simulink model "13_Solor_Charging_2W"  (R2024a)
settings: Solver=ode23t  StartTime=0.0  StopTime=3600  RelTol=1e-3
undefined symbols (not defined in the file): Ion, Lithium
libraries: spsDiodeLib x2, spsBatteryLib x1, spsSeriesRLCBranchLib x1, spsBoostConverterLib x1, spsParallelRLCBranchLib x1, spsPVArrayLib x1, spspowerguiLib x1
(part 2 of 2)

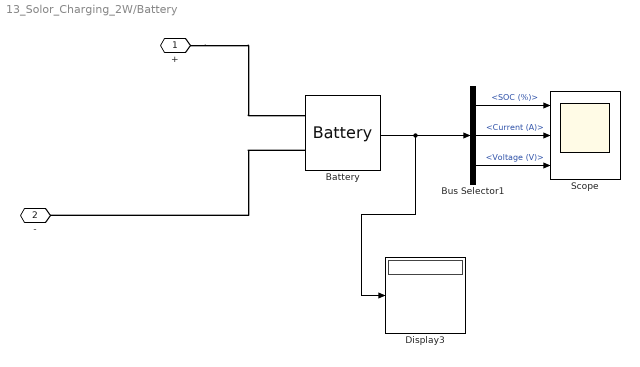
== system 13_Solor_Charging_2W/Battery ==
  Battery : spsBatteryLib/Battery  BatType=Lithium-Ion  ShowTempParam=off  ThermalPreset=no  ShowAgeParam=off  NomV=48  NomQ=65  SOC=25  Batt_Tr=30  PresetModel=on  MaxQ=65  MinV=36  FullV=55.8714  Dis_rate=28.2609  R=0.0073846  Normal_OP=58.7826  expZone="[51.8585      3.19348]"  current=[6.5 13 32.5]  Units=Time  Tci=20  NomT=20  T2=-30  MaxQ2=4.8  FullV2=7.1  Normal_OP2=5.655  expZone2="[6.58           1]"  Rca=0.6  ti=2000  Dp=0  Neq0=0  Tsim=1e6  Ta1=25  Qeol=5.4*0.9  Reol=0.013333*1.2  Char_age=[2.3478, 3]  Dis_age=[2.3478, 10]  N1=1500  N2=10500  N3=1000  N4=1400  Ta2=45  N5=950
  Bus Selector1 : BusSelector  OutputSignals=SOC (%),Current (A),Voltage (V)
  Display3 : Display
  Scope : Scope  NumInputPorts=3
  + : PMIOPort  Side=Left
  - : PMIOPort  Port=2  Side=Left
  wires:
  Bus Selector1/1 -> Scope/1  "<SOC (%)>"
  Battery/1 -> Display3/1, Bus Selector1/1
  Bus Selector1/3 -> Scope/3  "<Voltage (V)>"
  Bus Selector1/2 -> Scope/2  "<Current (A)>"
  connections:
  +/RConn1 -- Battery/LConn1
  Battery/LConn2 -- -/RConn1

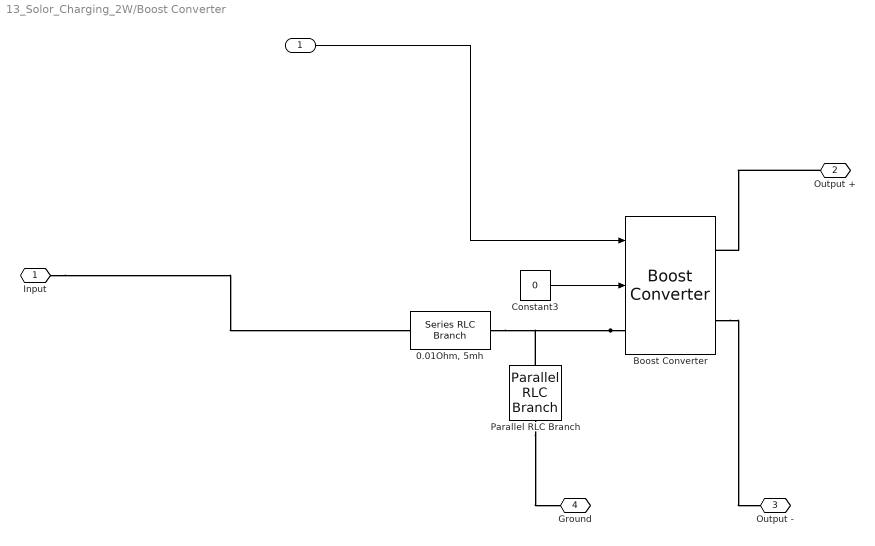
== system 13_Solor_Charging_2W/Boost Converter ==
  "  " : Inport
  "0.01Ohm, 5mh" : spsSeriesRLCBranchLib/Series RLC Branch  LConnTagsString=__new0  RConnTagsString=__new0  BranchType=RL  Resistance=0.0001  Inductance=1e-3  SetiL0=off  InitialCurrent=0  Capacitance=1e-6  Setx0=off  InitialVoltage=0  Measurements=None
  Boost Converter : spsBoostConverterLib/Boost Converter  ModelType=Switching function  Ron=1e-3  Rs=1e6  Cs=inf  Vforward=[0,0]  Ron_Diode=1e-3  Rs_Diode=1e6  Cs_Diode=inf  Vf_Diode=1e-3  Rs_CurrentSource=inf  Ron_ACsource=1e-3
      settings: LibrarySourceBlock=sps_lib/Power Electronics/Boost Converter
  Constant3 : Constant  Value=0
  Parallel RLC Branch : spsParallelRLCBranchLib/Parallel RLC Branch  LConnTagsString=a  RConnTagsString=__new0  BranchType=C  Resistance=1  Inductance=1e-3  SetiL0=off  InitialCurrent=0  Capacitance=100e-6  Setx0=off  InitialVoltage=0  Measurements=None
  Input : PMIOPort  Side=Left
  Output + : PMIOPort  Port=2  Side=Right
  Output - : PMIOPort  Port=3  Side=Right
  Ground : PMIOPort  Port=4  Side=Right
  wires:
  "  "/1 -> Boost Converter/1
  Constant3/1 -> Boost Converter/2
  connections:
  Input/RConn1 -- "0.01Ohm, 5mh"/LConn1
  Boost Converter/LConn1 -- "0.01Ohm, 5mh"/RConn1 -- Parallel RLC Branch/LConn1
  Output +/RConn1 -- Boost Converter/RConn1
  Parallel RLC Branch/RConn1 -- Ground/RConn1
  Boost Converter/RConn2 -- Output -/RConn1

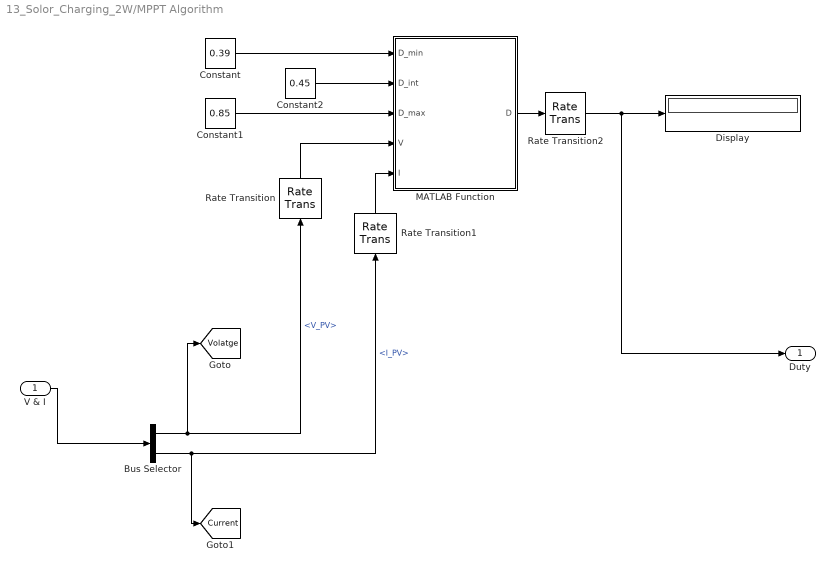
== system 13_Solor_Charging_2W/MPPT Algorithm ==
  V & I : Inport
  Bus Selector : BusSelector  OutputSignals=V_PV,I_PV
  Constant : Constant  Value=0.39
  Constant1 : Constant  Value=0.85
  Constant2 : Constant  Value=0.45
  Display : Display
  MATLAB Function : MATLAB Function  TreatAsAtomicUnit=on
  Rate Transition : RateTransition  OutPortSampleTime=0.0001
  Rate Transition1 : RateTransition  OutPortSampleTime=0.0001
  Rate Transition2 : RateTransition  OutPortSampleTime=5e-5
  Duty : Outport
  tag scope: Current=global, Volatge=global
  wires:
  Constant1/1 -> MATLAB Function/3(D_max)
  Rate Transition2/1 -> Duty/1, Display/1
  Rate Transition/1 -> MATLAB Function/4(V)
  Constant/1 -> MATLAB Function/1(D_min)
  Constant2/1 -> MATLAB Function/2(D_int)
  Rate Transition1/1 -> MATLAB Function/5(I)
  MATLAB Function/1(D) -> Rate Transition2/1
  Bus Selector/2 -> [Current], Rate Transition1/1  "<I_PV>"
  Bus Selector/1 -> [Volatge], Rate Transition/1  "<V_PV>"
  V & I/1 -> Bus Selector/1

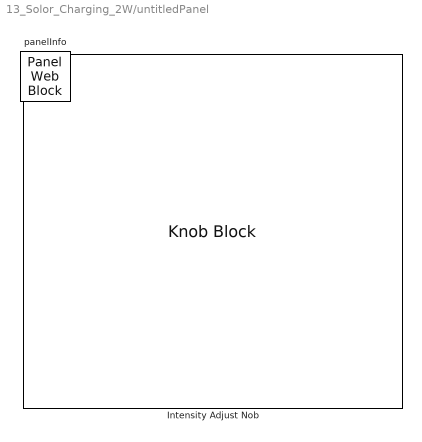
== system 13_Solor_Charging_2W/untitledPanel ==
  Intensity Adjust Nob : KnobBlock  Tag=HiddenForWebPanel  PanelInfo="{\"height\":354,\"left\":18,\"panelId\":\"panelId-075bc4ff-4528-4aae-9883-01d69de20ba9\",\"top\":18,\"type\":\"panelChild\",\"version\":\"2019b\",\"width\":379,\"zIndex\":1499998}"  LabelPosition=Hide  ScaleMax=1000
  panelInfo : PanelWebBlock  Tag=HiddenForWebPanel  PanelInfo="{\"compacted\":true,\"height\":394,\"isActiveTab\":true,\"left\":847,\"name\":\"Panel\",\"panelId\":\"panelId-075bc4ff-4528-4aae-9883-01d69de20ba9\",\"popoutData\":{\"height\":656,\"left\":1233,\"maximized\":false,\"top\":132,\"width\":303},\"popoutMode\":\"windowHidden\",\"tabIndex\":0,\"tabbedSetId\":\"tabbedSet1264567104\",\"top\":100,\"type\":\"panel\",\"version\":\"2019b\",\"visible\":true,\"width\":419,\"zIndex\":1500002}"  PanelSnapshot=<binary blob, 52036 chars, not shown>

== matlab function 13_Solor_Charging_2W/MPPT Algorithm/MATLAB Function ==
  data: D_min input; D_int input; D_max input; V input; I input; D output
function D = fcn(D_min, D_int, D_max, V, I)

D_const = 0.0015;

persistent  old_voltage old_power old_duty;

dataType = 'double';

if isempty(old_voltage)
    old_power = 0;
    old_voltage = 0;
    old_duty = D_int;
end

Updated_Voltage = old_voltage;

% Find power
N_power = V * I;

if (N_power ~= old_power)

    % Find Max power and volatge
    if (N_power > old_power)
        old_power = N_power;

        %increase the Vref
        if((V < Updated_Voltage) && (old_duty>D_min) && (old_duty<D_max))

            old_duty = old_duty + D_const;

            %decrease the Vref
        elseif (old_duty>D_min && old_duty<D_max)

            old_voltage = V;
            old_duty = old_duty - D_const;
        end

    else
        %increase the Vref
        if((V < Updated_Voltage) && (old_duty>D_min) && (old_duty<D_max))

            old_duty = old_duty - D_const;

            %decrease the Vref
        elseif (old_duty>D_min && old_duty<D_max)

            old_voltage = V;
            old_duty = old_duty + D_const;
        end
    end
    D = old_duty;
else
    D = old_duty;
end
